simulink model "PID_Controller"  (R2021a)
settings: Solver=ode45  StartTime=0.0  StopTime=10.0  RelTol=1e-3
settings Model: Creator=sansh  LastModifiedBy=TitusChoi
settings SolverCC: AlgebraicLoopSolver=TrustRegion
settings DataIOCC: ReturnWorkspaceOutputs=off
settings DebuggingCC: SFMachineParentedDataDiag=warning  ArithmeticOperatorsInVariantConditions=warning
settings SFSimCC: SimUseLocalCustomCode=off  CustomCodeUndefinedFunction=UseInterfaceOnly
settings RTWCC: RTWUseLocalCustomCode=off
settings CodeAppCC: StateflowObjectComments=on

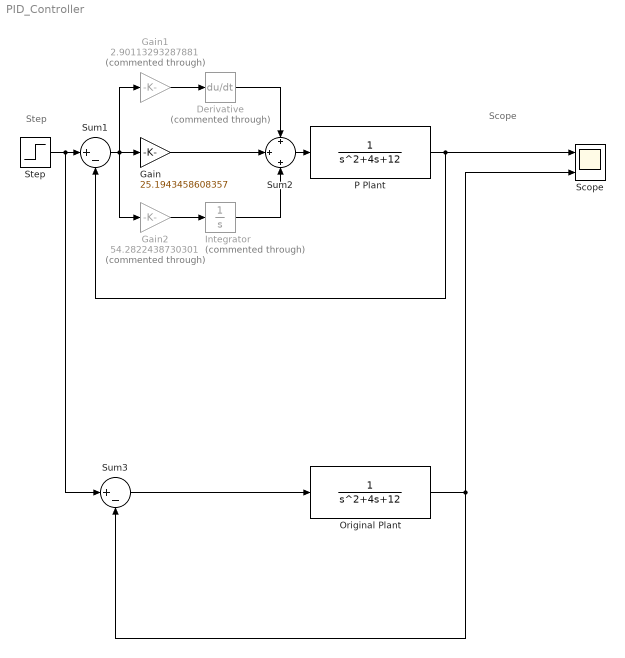
== system PID_Controller ==
  note: Step
  note: Scope
  Derivative : Derivative  Commented=through
  Gain : Gain  Gain=25.1943458608357
  Gain1 : Gain  Commented=through  Gain=2.90113293287881
  Gain2 : Gain  Commented=through  Gain=54.2822438730301
  Integrator : Integrator  Commented=through
  Original Plant : TransferFcn  Denominator=[1 4 12]
  P Plant : TransferFcn  Denominator=[1 4 12]
  Scope : Scope  NumInputPorts=2
  Step : Step  SampleTime=0
  Sum1 : Sum  Inputs=|+-
  Sum2 : Sum  Inputs=+|+|+
  Sum3 : Sum  Inputs=|+-
  wires:
  P Plant/1 -> Sum1/2, Scope/1
  Sum1/1 -> Gain/1, Gain2/1, Gain1/1
  Gain1/1 -> Derivative/1
  Gain2/1 -> Integrator/1
  Gain/1 -> Sum2/2
  Sum2/1 -> P Plant/1
  Integrator/1 -> Sum2/3
  Derivative/1 -> Sum2/1
  Original Plant/1 -> Sum3/2, Scope/2
  Step/1 -> Sum3/1, Sum1/1
  Sum3/1 -> Original Plant/1
